simulink model "Multiplexer_simulink"  (R2018a)
settings: Solver=FixedStepAuto  StartTime=0.0  StopTime=050  FixedStep=1  RelTol=1e-3
libraries: fl_lib x14, nesl_utility x6
settings Model: Creator=Kalindi  LastModifiedBy=Kalindi

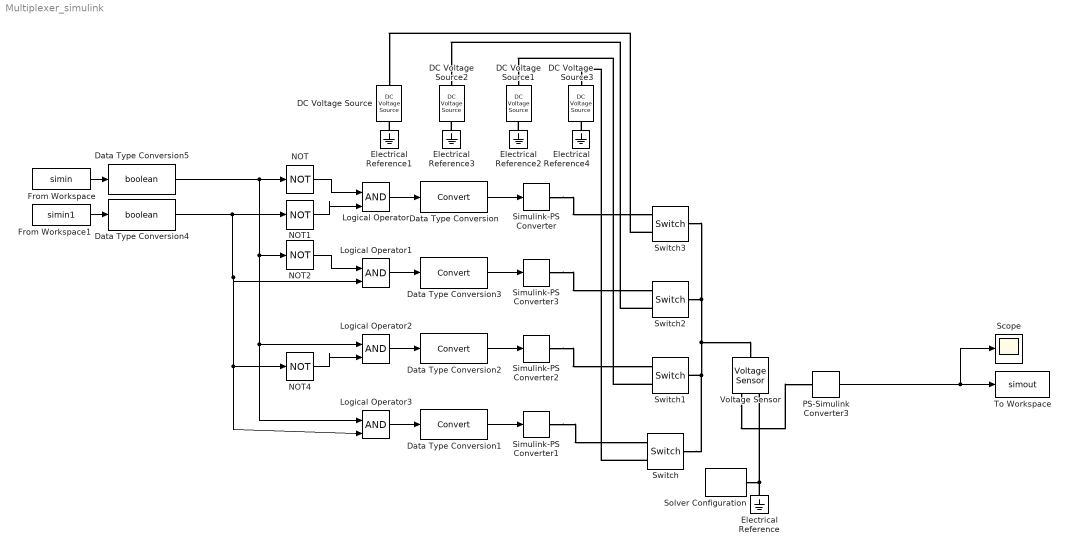
== system Multiplexer_simulink ==
  DC Voltage Source : fl_lib/Electrical/Electrical Sources/DC Voltage Source  v0=1 V
  DC Voltage Source1 : fl_lib/Electrical/Electrical Sources/DC Voltage Source  v0=3 V
  DC Voltage Source2 : fl_lib/Electrical/Electrical Sources/DC Voltage Source  v0=2 V
  DC Voltage Source3 : fl_lib/Electrical/Electrical Sources/DC Voltage Source  v0=4 V
  Data Type Conversion{,1..3} (4 alike) : DataTypeConversion
  Data Type Conversion4 : DataTypeConversion  OutDataTypeStr=boolean
  Data Type Conversion5 : DataTypeConversion  OutDataTypeStr=boolean
  Electrical Reference{,1..4} (5 alike) : fl_lib/Electrical/Electrical Elements/Electrical Reference
  From Workspace : FromWorkspace  VariableName=simin
  From Workspace1 : FromWorkspace  VariableName=simin1
  Logical Operator{,1..3} (4 alike) : Logic  IconShape=distinctive  AllPortsSameDT=off  OutDataTypeStr=boolean
  NOT{,1..2,4} (4 alike) : Logic  Operator=NOT  IconShape=distinctive  AllPortsSameDT=off  OutDataTypeStr=boolean
  PS-Simulink Converter3 : nesl_utility/PS-Simulink Converter  PhysicalDomain=network_engine_domain  SubClassName=ps_output  LeftPortType=input  RightPortType=output  PseudoPeriodic=off  Frequencies=[]  Unit=1  AffineConversion=off
  Scope : Scope
  Simulink-PS Converter{,1..3} (4 alike) : nesl_utility/Simulink-PS Converter  PhysicalDomain=network_engine_domain  SubClassName=ps_input  LeftPortType=input  RightPortType=output  PseudoPeriodic=off  Frequencies=[]  NoiseDistribution=none  NoiseParameters=[]  Unit=V  AffineConversion=off  FilteringAndDerivatives=provide  SimscapeFilterOrder=1  InputFilterTimeConstant=0.001  UdotUserProvided=0
  Solver Configuration : nesl_utility/Solver Configuration  PhysicalDomain=network_engine_domain  SubClassName=solver  LeftPortType=input  RightPortType=generic  Tones=[]  Harmonics=[]  SimulateNoise=off  Profile=off  UseLocalSampling=off  EnableSwitchedLinearOptims=on  FrequencyDomain=off  UseCCode=off  RelTol=0.001  AbsTol=1e-06  MinStep=1e-09  ToWorkspace=off  RevertToSquareIcSolve=off  NumHomotopyIterations=100  PhasorMode=off  PhasorModeNumHarmonics=1  DoDC=off  ResidualTolerance=1e-09  UseLocalSolver=off  LocalSolverChoice=NE_BACKWARD_EULER_ADVANCER  LocalSolverSampleTime=0.001  DoFixedCost=off  MaxNonlinIter=3  MaxModeIter=2  LinearAlgebra=Sparse  EquationFormulation=NE_TIME_EF  DelaysMemoryBudget=1024  AutomaticFiltering=on  FilteringTimeConstant=0.001
  Switch{,1..3} (4 alike) : fl_lib/Electrical/Electrical Elements/Switch  R_closed=0.01 Ohm  G_open=1e-8 1/Ohm  Threshold=.5  i_specify=off  i_priority=None  i=0 A  i_nominal_specify=off  i_nominal_unit=A  i_nominal_value=1  v_specify=off  v_priority=None  v=0 V  v_nominal_specify=off  v_nominal_unit=V  v_nominal_value=1
      settings: SourceProductName=Simscape
  To Workspace : ToWorkspace  VariableName=simout  SaveFormat=Timeseries  SampleTime=-1
  Voltage Sensor : fl_lib/Electrical/Electrical Sensors/Voltage Sensor
  wires:
  NOT/1 -> Logical Operator/1
  NOT1/1 -> Logical Operator/2
  PS-Simulink Converter3/1 -> Scope/1, To Workspace/1
  NOT2/1 -> Logical Operator1/1
  NOT4/1 -> Logical Operator2/2
  Logical Operator/1 -> Data Type Conversion/1
  Data Type Conversion/1 -> Simulink-PS Converter/1
  Data Type Conversion3/1 -> Simulink-PS Converter3/1
  Logical Operator2/1 -> Data Type Conversion2/1
  Logical Operator3/1 -> Data Type Conversion1/1
  Data Type Conversion1/1 -> Simulink-PS Converter1/1
  Data Type Conversion2/1 -> Simulink-PS Converter2/1
  Logical Operator1/1 -> Data Type Conversion3/1
  From Workspace1/1 -> Data Type Conversion4/1
  From Workspace/1 -> Data Type Conversion5/1
  Data Type Conversion4/1 -> Logical Operator3/2, NOT4/1, Logical Operator1/2, NOT1/1
  Data Type Conversion5/1 -> NOT/1, Logical Operator3/1, Logical Operator2/1, NOT2/1
  connections:
  Simulink-PS Converter/RConn1 -- Switch3/RConn1
  Electrical Reference/LConn1 -- Solver Configuration/RConn1 -- Voltage Sensor/RConn2
  Simulink-PS Converter3/RConn1 -- Switch2/RConn1
  Simulink-PS Converter2/RConn1 -- Switch1/RConn1
  Simulink-PS Converter1/RConn1 -- Switch/RConn1
  Electrical Reference2/LConn1 -- DC Voltage Source1/RConn1
  Electrical Reference3/LConn1 -- DC Voltage Source2/RConn1
  Electrical Reference1/LConn1 -- DC Voltage Source/RConn1
  Electrical Reference4/LConn1 -- DC Voltage Source3/RConn1
  Switch3/RConn2 -- DC Voltage Source/LConn1
  Switch2/RConn2 -- DC Voltage Source2/LConn1
  Switch1/RConn2 -- DC Voltage Source1/LConn1
  Switch/RConn2 -- DC Voltage Source3/LConn1
  Voltage Sensor/RConn1 -- PS-Simulink Converter3/LConn1
  Switch3/LConn1 -- Switch/LConn1 -- Switch1/LConn1 -- Voltage Sensor/LConn1 -- Switch2/LConn1
